simulink model "DynamicControl"  (R2015a)
settings: Solver=ode5  StartTime=0.0  StopTime=15  FixedStep=0.001  RelTol=1e-3
values from neighbouring files (symbols this model uses):
  Kp = 25    [Init.m]
  Kv = 10    [Init.m]
  L = 0.13    [Init.m]    (also in KinematicPlot.m; plotVehicle.m)
  L_e = (1 + err_L)*L    (= 0.13)    [Init.m]
  r = 0.1    [Init.m]    (also in KinematicPlot.m)
  R = 2    [Init.m]
  r_e = (1 + err_r)*r    (= 0.1)    [Init.m]
  theta0 = pi    (= 3.14159265359)    [Init.m]
  wd = 0.5    [Init.m]
  x0 = 2.3    [Init.m]
  y0 = 0    [Init.m]
undefined symbols (not defined in the file): d
settings Model: Creator=tgvo  LastModifiedBy=tgvo
settings DataIOCC: LimitDataPoints=off
settings DebuggingCC: AlgebraicLoopMsg=none

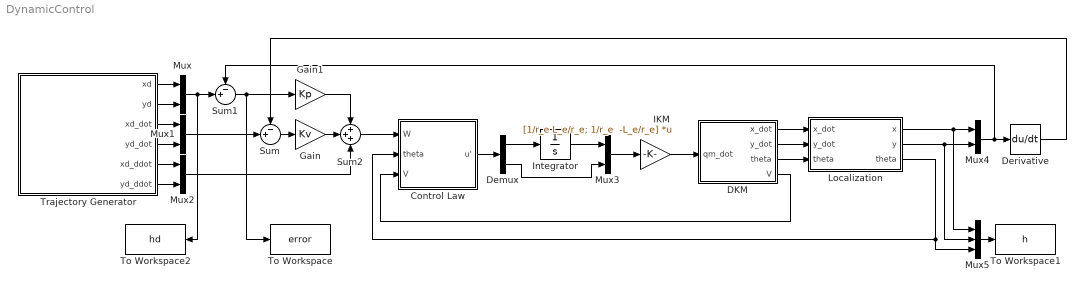
== system DynamicControl ==
  Control Law : Subsystem
  DKM : Subsystem  mask{r=r, L=L, theta0=theta0}
      mask prompts: r "Wheel Raidus (r)"; L "Half of Track Gauge (L)"; theta0 "Initial value of theta (theta0)"
  Demux : Demux  Outputs=2
  Derivative : Derivative
  Gain : Gain  Gain=Kv
  Gain1 : Gain  Gain=Kp
  IKM : Gain  Gain="[1/r_e L_e/r_e; 1/r_e  -L_e/r_e]"  Multiplication=Matrix(K*u) (u vector)
  Integrator : Integrator  InitialCondition=1
  Localization : Subsystem  mask{x0=x0, y0=y0, d=d}
      mask prompts: x0 "Initial value of x (x0)"; y0 "Initial value of y (y0)"; d "Distqnce b/w P and Om"
  Mux{,1..4} (5 alike) : Mux  Inputs=2
  Mux5 : Mux  Inputs=3
  Sum : Sum  Inputs=-+|
  Sum1 : Sum  Inputs=-+|
  Sum2 : Sum  Inputs=+++
  To Workspace : ToWorkspace  VariableName=error  SampleTime=-1
  To Workspace1 : ToWorkspace  VariableName=h  SampleTime=-1
  To Workspace2 : ToWorkspace  VariableName=hd  SampleTime=-1
  Trajectory Generator : Subsystem  mask{R=R, wd=wd}
      mask prompts: R "Trajectory Radius (R)"; wd "Desired Angular Velocity (wd)"
  wires:
  Trajectory Generator/1(xd) -> Mux/1
  Trajectory Generator/2(yd) -> Mux/2
  Trajectory Generator/4(yd_dot) -> Mux1/2
  Trajectory Generator/3(xd_dot) -> Mux1/1
  Trajectory Generator/6(yd_ddot) -> Mux2/2
  Trajectory Generator/5(xd_ddot) -> Mux2/1
  Mux1/1 -> Sum/2
  Sum/1 -> Gain/1
  Sum1/1 -> To Workspace/1, Gain1/1
  Mux/1 -> To Workspace2/1, Sum1/2
  Gain/1 -> Sum2/2
  Gain1/1 -> Sum2/1
  Mux2/1 -> Sum2/3
  Control Law/1(u') -> Demux/1
  Demux/1 -> Integrator/1
  Integrator/1 -> Mux3/1
  Demux/2 -> Mux3/2
  Mux3/1 -> IKM/1
  IKM/1 -> DKM/1(qm_dot)
  Localization/3(theta) -> Control Law/2(theta), Mux5/3
  Localization/1(x) -> Mux5/1, Mux4/1
  Localization/2(y) -> Mux5/2, Mux4/2
  Mux5/1 -> To Workspace1/1
  Mux4/1 -> Derivative/1, Sum1/1
  Derivative/1 -> Sum/1
  Sum2/1 -> Control Law/1(W)
  DKM/4(V) -> Control Law/3(V)
  DKM/1(x_dot) -> Localization/1(x_dot)
  DKM/2(y_dot) -> Localization/2(y_dot)
  DKM/3(theta) -> Localization/3("theta ")

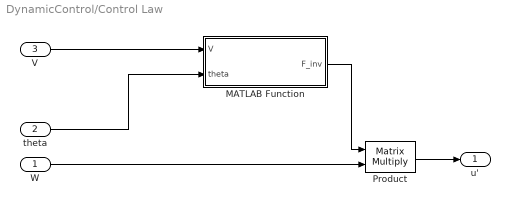
== system DynamicControl/Control Law ==
  W : Inport
  theta : Inport  Port=2
  V : Inport  Port=3
  MATLAB Function : MATLAB Function  TreatAsAtomicUnit=on
  Product : Product  Multiplication=Matrix(*)
  u' : Outport
  wires:
  W/1 -> Product/2
  Product/1 -> u'/1
  theta/1 -> MATLAB Function/2(theta)
  MATLAB Function/1(F_inv) -> Product/1
  V/1 -> MATLAB Function/1(V)

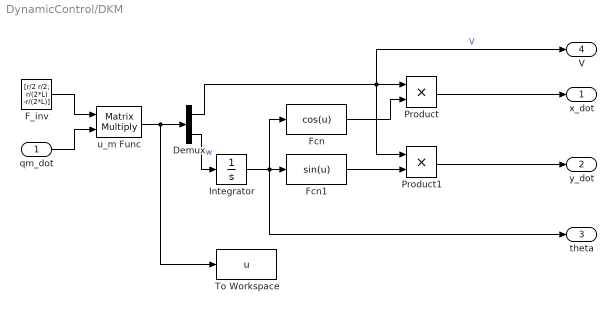
== system DynamicControl/DKM ==
  qm_dot : Inport
  Demux : Demux  Outputs=2
  F_inv : Constant  Value=[r/2 r/2; r/(2*L) -r/(2*L)]
  Fcn : Fcn  Expr=cos(u)
  Fcn1 : Fcn  Expr=sin(u)
  Integrator : Integrator  InitialCondition=theta0
  Product : Product
  Product1 : Product
  To Workspace : ToWorkspace  VariableName=u  SampleTime=-1
  u_m Func : Product  Multiplication=Matrix(*)
  x_dot : Outport
  y_dot : Outport  Port=2
  theta : Outport  Port=3
  V : Outport  Port=4
  wires:
  F_inv/1 -> u_m Func/1
  qm_dot/1 -> u_m Func/2
  Demux/2 -> Integrator/1  "w"
  u_m Func/1 -> To Workspace/1, Demux/1
  Fcn/1 -> Product/2
  Fcn1/1 -> Product1/2
  Integrator/1 -> theta/1, Fcn/1, Fcn1/1
  Demux/1 -> V/1, Product1/1, Product/1  "V"
  Product/1 -> x_dot/1
  Product1/1 -> y_dot/1

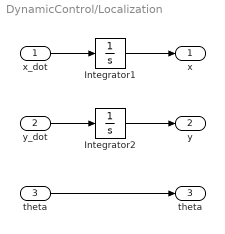
== system DynamicControl/Localization ==
  x_dot : Inport
  y_dot : Inport  Port=2
  "theta " : Inport  Port=3
  Integrator1 : Integrator  InitialCondition=x0
  Integrator2 : Integrator  InitialCondition=y0
  x : Outport
  y : Outport  Port=2
  theta : Outport  Port=3
  wires:
  Integrator1/1 -> x/1
  Integrator2/1 -> y/1
  x_dot/1 -> Integrator1/1
  y_dot/1 -> Integrator2/1
  "theta "/1 -> theta/1

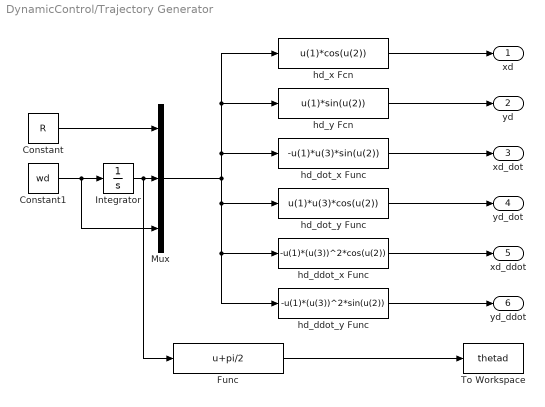
== system DynamicControl/Trajectory Generator ==
  Constant : Constant  Value=R
  Constant1 : Constant  Value=wd
  Func : Fcn  Expr=u+pi/2
  Integrator : Integrator
  Mux : Mux  Inputs=3
  To Workspace : ToWorkspace  VariableName=thetad  SampleTime=-1
  hd_ddot_x Func : Fcn  Expr=-u(1)*(u(3))^2*cos(u(2))
  hd_ddot_y Func : Fcn  Expr=-u(1)*(u(3))^2*sin(u(2))
  hd_dot_x Func : Fcn  Expr=-u(1)*u(3)*sin(u(2))
  hd_dot_y Func : Fcn  Expr=u(1)*u(3)*cos(u(2))
  hd_x Fcn : Fcn  Expr=u(1)*cos(u(2))
  hd_y Fcn : Fcn  Expr=u(1)*sin(u(2))
  xd : Outport
  yd : Outport  Port=2
  xd_dot : Outport  Port=3
  yd_dot : Outport  Port=4
  xd_ddot : Outport  Port=5
  yd_ddot : Outport  Port=6
  wires:
  hd_dot_x Func/1 -> xd_dot/1
  hd_ddot_y Func/1 -> yd_ddot/1
  hd_y Fcn/1 -> yd/1
  hd_x Fcn/1 -> xd/1
  Mux/1 -> hd_ddot_y Func/1, hd_ddot_x Func/1, hd_dot_y Func/1, hd_y Fcn/1, hd_x Fcn/1, hd_dot_x Func/1
  hd_dot_y Func/1 -> yd_dot/1
  hd_ddot_x Func/1 -> xd_ddot/1
  Constant1/1 -> Mux/3, Integrator/1
  Constant/1 -> Mux/1
  Integrator/1 -> Func/1, Mux/2
  Func/1 -> To Workspace/1

== matlab function DynamicControl/Control Law/MATLAB Function ==
  data: V input; F_inv output; theta input
function F_inv = Find_F_inv(V,theta)

F_inv = inv([cos(theta) -V*sin(theta);sin(theta) V*cos(theta)]);

end
